simulink model "Four_V_by_f_Ctrl_VFD"  (R2024a)
settings: Solver=ode23tb  StartTime=0.0  StopTime=5  MaxStep=1e-4  RelTol=1e-3  EnableMultiTasking=on
libraries: spsIGBTDiodeLib x6, spsSawtoothGeneratorLib x3, simulink x2, spsAsynchronousMachineSIUnitsLib x1, spsVoltageMeasurementLib x1, spsDCVoltageSourceLib x1, sps_lib x1
settings Model: Creator=Amr Saleh  LastModifiedBy=91889
settings SolverCC: AlgebraicLoopSolver=TrustRegion
settings DataIOCC: LimitDataPoints=on  SaveFormat=Array  ReturnWorkspaceOutputs=off
settings OptimizationCC: LifeSpan=inf
settings DebuggingCC: SolverPrmCheckMsg=warning  UnconnectedInputMsg=warning  UnconnectedOutputMsg=warning  UnconnectedLineMsg=warning  SFUnexpectedBacktrackingDiag=warning  SFNoUnconditionalDefaultTransitionDiag=warning  SFExecutionAtInitializationDiag=none  ArithmeticOperatorsInVariantConditions=warning
settings HardwareCC: ProdBitPerPointer=32  ProdBitPerSizeT=32  ProdBitPerPtrDiffT=32  ProdLargestAtomicFloat=None  ProdIntDivRoundTo=Undefined  ProdEndianess=Unspecified  ProdWordSize=32  ProdHWDeviceType=32-bit Generic
settings ModelReferenceCC: PropagateSignalLabelsOutOfModel=off
settings SFSimCC: SimUseLocalCustomCode=off  CustomCodeUndefinedFunction=UseInterfaceOnly
settings RTWCC: RTWUseLocalCustomCode=off  GPUComputeCapability=3.5
settings CodeAppCC: StateflowObjectComments=on
settings GRTTargetCC: TargetLangStandard=C89/C90 (ANSI)
settings ConfigComp: CovMetricSettings=dw  CovSaveCumulativeToWorkspaceVar=on  CovSaveSingleToWorkspaceVar=on  CovExternalEMLEnable=off  CovSFcnEnable=off
settings SimscapeCC: SimscapeNormalizeSystem=off

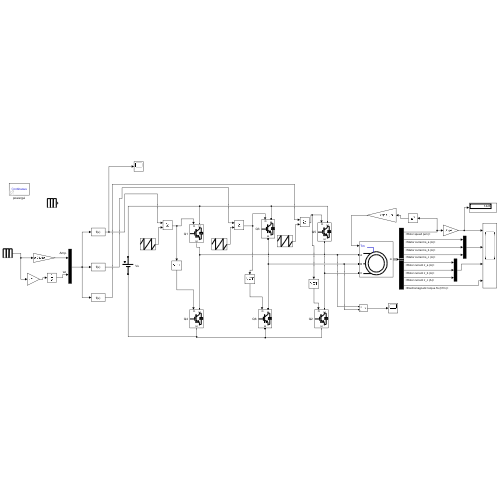
[thumbnail: Simulink's stored preview of the top-level diagram]
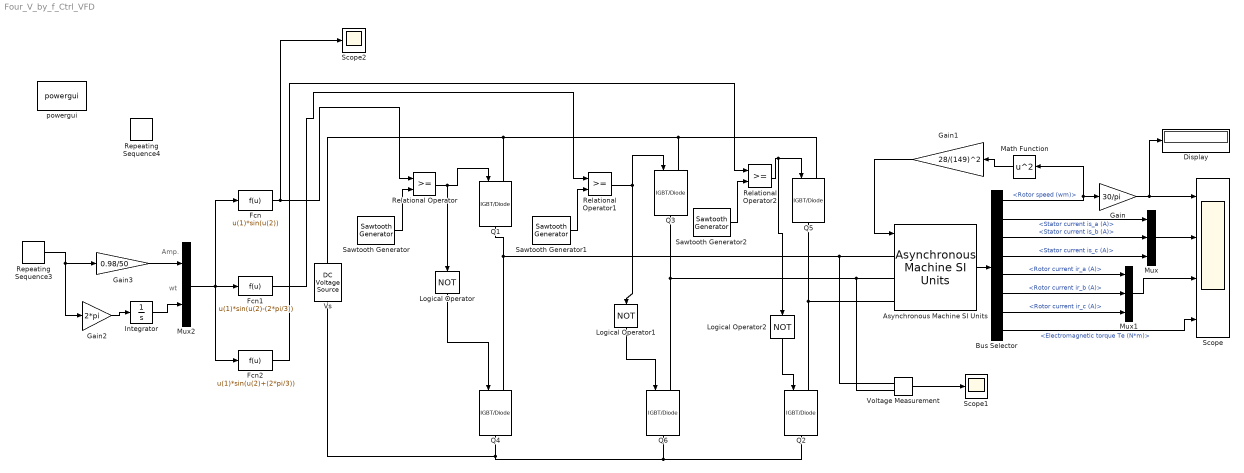
== system Four_V_by_f_Ctrl_VFD ==
  note: wt
  note: Amp.
  Asynchronous Machine SI Units : spsAsynchronousMachineSIUnitsLib/Asynchronous Machine SI Units  RotorType=Squirrel-cage  PresetModel="15:  5.4 HP (4KW)   400 V  50Hz 1430 RPM"  MechanicalLoad=Torque Tm  ShowDetailedParameters=on  ReferenceFrame=Rotor  Units=SI  MeasurementBus=off  NominalParameters=[4000 400 50]  VoltageRatio=1  Stator=[1.405 0.005839]  Rotor=[1.395 0.005839]  Cage1=[ 0.022 0.226/377]  Cage2=[ 0.022 0.226/377]  Lm=0.1722  Mechanical=[0.0131 0.002985 2]  PolePairs=2  InitialConditions=[1 0 0 0 0 0 0 0]  SimulateSaturation=off  Saturation=[14.03593122, 27.81365428, 53.79336849, 72.68890987, 97.98006896, 148.6815601, 215.7428561, 302.9841135, 420.4778367 ; 230, 322, 414, 460, 506, 552, 598, 644, 690]  LoadFlowParameters=1492000  TsPowergui=0  TsBlock=-1  IterativeModel=Trapezoidal non iterative  IterativeDiscreteModel=Trapezoidal non iterative  Pmec=0
      settings: AttributesFormatString=\n
  Bus Selector : BusSelector  OutputSignals=Mechanical.Rotor speed (wm),Stator measurements.Stator current is_a (A),Stator measurements.Stator current is_b (A),Stator measurements.Stator current is_c (A),Rotor measurements.Rotor current ir_a (A),Rotor measurements.Rotor current ir_b (A),Rotor measurements.Rotor current ir_c (A),Mechanical.Electromagnetic torque Te (N*m)
  Display : Display
  Fcn : Fcn  Expr=u(1)*sin(u(2))
  Fcn1 : Fcn  Expr=u(1)*sin(u(2)-(2*pi/3))
  Fcn2 : Fcn  Expr=u(1)*sin(u(2)+(2*pi/3))
  Gain : Gain  Gain=30/pi
  Gain1 : Gain  Gain=28/(149)^2
  Gain2 : Gain  Gain=2*pi
  Gain3 : Gain  Gain=0.98/50
  Integrator : Integrator
  Logical Operator : Logic  Operator=NOT  AllPortsSameDT=off  OutDataTypeStr=boolean
  Logical Operator1 : Logic  Operator=NOT  AllPortsSameDT=off  OutDataTypeStr=boolean
  Logical Operator2 : Logic  Operator=NOT  AllPortsSameDT=off  OutDataTypeStr=boolean
  Math Function : Math  Operator=square  SignedPower=on
  Mux : Mux  Inputs=3
  Mux1 : Mux  Inputs=3
  Mux2 : Mux  Inputs=2
  Q{1..6} (6 alike) : spsIGBTDiodeLib/IGBT//Diode  Ron=1e-3  Rs=1e5  Cs=inf  Measurements=off
  Relational Operator : RelationalOperator  OutDataTypeStr=boolean  InputSameDT=off
  Relational Operator1 : RelationalOperator  OutDataTypeStr=boolean  InputSameDT=off
  Relational Operator2 : RelationalOperator  OutDataTypeStr=boolean  InputSameDT=off
  Repeating Sequence3 : simulink/Sources/Repeating Sequence  rep_seq_t=[0 0.2 10]  rep_seq_y=[0 50 50]
  Repeating Sequence4 : simulink/Sources/Repeating Sequence  rep_seq_t=[0 0.2 10]  rep_seq_y=[0 50 50]
  Sawtooth Generator : spsSawtoothGeneratorLib/Sawtooth Generator  Freq=1000  Phase=180  Ts=0
  Sawtooth Generator1 : spsSawtoothGeneratorLib/Sawtooth Generator  Freq=1000  Phase=180  Ts=0
  Sawtooth Generator2 : spsSawtoothGeneratorLib/Sawtooth Generator  Freq=1000  Phase=180  Ts=0
  Scope : Scope  NumInputPorts=4
  Scope1 : Scope
  Scope2 : Scope
  Voltage Measurement : spsVoltageMeasurementLib/Voltage Measurement  PhasorSimulation=off  OutputType=Complex  PSBequivalent=0
  Vs : spsDCVoltageSourceLib/DC Voltage Source  Amplitude=650  Measurements=None
  powergui : sps_lib/powergui  Priority=1  SimulationMode=Continuous  SampleTime=50e-6  frequency=60  Iterations=50  frequencyindice=50  Pbase=100e6  ErrMax=1e-4  UnitsV=kV  UnitsW=MW  buscounter=0  FunctionMessages=off  echomessages=off  EnableUseOfTLC=off  CurrentSourceSwitches=off  DisableSnubberDevices=off  DisableRonSwitches=off  DisableVfSwitches=off  DisplayEquations=off  AutomaticDiscreteSolvers=off  SolverType=Tustin/Backward Euler (TBE)  Interpol=off  ExternalGateDelay=off  methode=off  Ts=100  x0status=blocks  SPID=off  SwTol=0  HookPort=off  NonlinearTolerance=1e-4  nMaxIteration=100  ContinueOnMaxIteration=off  RestoreLinks=warning  ResistiveCurrentMeasurement=off  Frange=[0:2:500]  Ylog=off  Xlog=on  ShowGrid=off  save=off  variable=ZData  structure=0  ZoomFFT=off  StartTime=0.0  cycles=1  DisplayStyle=1  fundamental=60  FreqAxis=off  MaxFrequency=1000  frequencyindicesteady=1  RmsSteady=1  display=off
  wires:
  Gain1/1 -> Asynchronous Machine SI Units/1
  Asynchronous Machine SI Units/1 -> Bus Selector/1
  Bus Selector/2 -> Mux/1  "<Stator current is_a (A)>"
  Bus Selector/3 -> Mux/2  "<Stator current is_b (A)>"
  Bus Selector/4 -> Mux/3  "<Stator current is_c (A)>"
  Bus Selector/6 -> Mux1/2  "<Rotor current ir_b (A)>"
  Bus Selector/7 -> Mux1/3  "<Rotor current ir_c (A)>"
  Bus Selector/5 -> Mux1/1  "<Rotor current ir_a (A)>"
  Bus Selector/1 -> Math Function/1, Gain/1  "<Rotor speed (wm)>"
  Bus Selector/8 -> Scope/4  "<Electromagnetic torque Te (N*m)>"
  Mux/1 -> Scope/2
  Mux1/1 -> Scope/3
  Gain/1 -> Display/1, Scope/1
  Math Function/1 -> Gain1/1
  Mux2/1 -> Fcn/1, Fcn1/1, Fcn2/1
  Repeating Sequence3/1 -> Gain2/1, Gain3/1
  Gain2/1 -> Integrator/1
  Integrator/1 -> Mux2/2
  Fcn/1 -> Scope2/1, Relational Operator/1
  Sawtooth Generator/1 -> Relational Operator/2
  Relational Operator/1 -> Q1/1, Logical Operator/1
  Fcn1/1 -> Relational Operator1/1
  Sawtooth Generator1/1 -> Relational Operator1/2
  Fcn2/1 -> Relational Operator2/1
  Sawtooth Generator2/1 -> Relational Operator2/2
  Relational Operator2/1 -> Q5/1, Logical Operator2/1
  Logical Operator/1 -> Q4/1
  Logical Operator1/1 -> Q6/1
  Relational Operator1/1 -> Q3/1, Logical Operator1/1
  Logical Operator2/1 -> Q2/1
  Voltage Measurement/1 -> Scope1/1
  Gain3/1 -> Mux2/1
  connections:
  Q3/LConn1 -- Q5/LConn1 -- Vs/RConn1 -- Q1/LConn1
  Q5/RConn1 -- Asynchronous Machine SI Units/LConn3 -- Q2/LConn1
  Q3/RConn1 -- Q6/LConn1 -- Voltage Measurement/LConn2 -- Asynchronous Machine SI Units/LConn2
  Q4/LConn1 -- Q1/RConn1 -- Voltage Measurement/LConn1 -- Asynchronous Machine SI Units/LConn1
  Q2/RConn1 -- Q6/RConn1 -- Q4/RConn1 -- Vs/LConn1
